simulink model "audio"  (R2018b)
settings: Solver=VariableStepAuto  StartTime=0.0  StopTime=0.2  RelTol=1e-3
settings Model: Creator=caeuser  LastModifiedBy=caeuser
settings OptimizationCC: BlockReduction=off  ConditionallyExecuteInputs=off  DefaultParameterBehavior=Inlined
settings DebuggingCC: AlgebraicLoopMsg=error
settings HardwareCC: ProdBitPerPointer=32  ProdBitPerSizeT=32  ProdBitPerPtrDiffT=32  ProdLargestAtomicFloat=None  ProdIntDivRoundTo=Undefined  ProdEndianess=Unspecified  ProdWordSize=32  ProdHWDeviceType=ASIC/FPGA->ASIC/FPGA  TargetBitPerLong=64  TargetBitPerPointer=64  TargetBitPerSizeT=64  TargetBitPerPtrDiffT=64  TargetLongLongMode=on  TargetIntDivRoundTo=Zero  TargetEndianess=LittleEndian  TargetWordSize=64  TargetHWDeviceType=Custom Processor->MATLAB Host Computer  ProdEqTarget=off

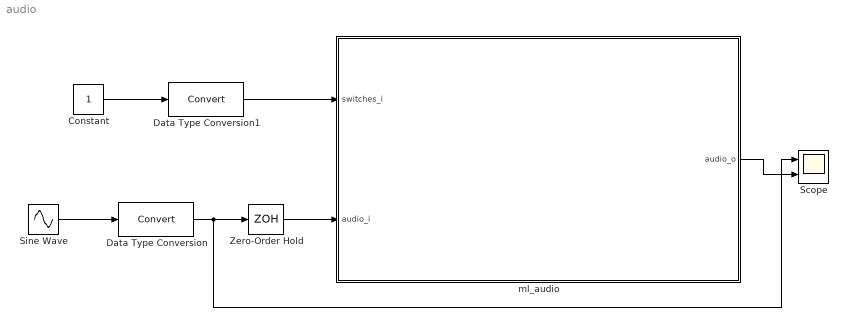
== system audio ==
  Constant : Constant  SampleTime=1/48000
  Data Type Conversion : DataTypeConversion
  Data Type Conversion1 : DataTypeConversion  SaturateOnIntegerOverflow=on
  Scope : Scope  NumInputPorts=2
  Sine Wave : Sin  Amplitude=0.9  Frequency=2*3.14*1500  SampleTime=0
  Zero-Order Hold : ZeroOrderHold  SampleTime=1/48000
  ml_audio : Subsystem
  wires:
  Constant/1 -> Data Type Conversion1/1
  Data Type Conversion/1 -> Zero-Order Hold/1, Scope/1
  Data Type Conversion1/1 -> ml_audio/1(switches_i)
  ml_audio/1(audio_o) -> Scope/2
  Zero-Order Hold/1 -> ml_audio/2(audio_i)
  Sine Wave/1 -> Data Type Conversion/1

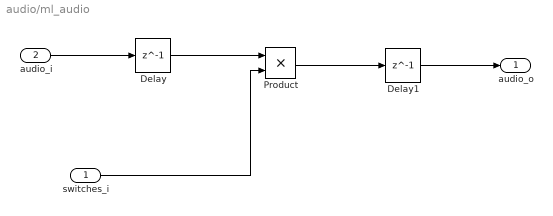
== system audio/ml_audio ==
  switches_i : Inport  OutDataTypeStr=fixdt(0,10,10)
  audio_i : Inport  Port=2  OutDataTypeStr=fixdt(1,16,15)
  Delay : Delay  DelayLength=1  InitialCondition=0
  Delay1 : Delay  DelayLength=1  InitialCondition=0
  Product : Product  OutDataTypeStr=fixdt(1,16,15)
  audio_o : Outport  OutDataTypeStr=fixdt(1,16,15)
  wires:
  audio_i/1 -> Delay/1
  Delay1/1 -> audio_o/1
  Delay/1 -> Product/1
  Product/1 -> Delay1/1
  switches_i/1 -> Product/2
